simulink model "Discrete_Time_Sim_With_Noise"  (R2024b)
settings: Solver=FixedStepAuto  StartTime=0.0  StopTime=10  FixedStep=0.001  RelTol=1e-3
undefined symbols (not defined in the file or in its folder): DiscIntNeverNeededParam, dspblkCoreblockFVToolHelper, gcbh
libraries: simulink x12, sharedTrackingLibrary x1
(part 3 of 4)

== matlab function Discrete_Time_Sim_With_Noise/PLANT/MATLAB Function ==
  data: F1 input; D2_THETA_1 output; F2 input; F3 input; F4 input; F5 input; F6 input; states input; D2_THETA_2 output; D2_THETA_3 output
function [D2_THETA_1, D2_THETA_2, D2_THETA_3]  = fcn(F1, F2, F3, F4, F5, F6, states)

theta1 = states(1);
theta2 = states(2);
theta3 = states(3);
D_THETA_1 = states(4);
D_THETA_2 = states(5);
D_THETA_3 = states(6);

D2_THETA_1 =  (-1.539e-5*(D_THETA_1^2)*sin(theta3) - 1.71e-5*(D_THETA_1^2)*sin(theta2 + theta3) - 3.078e-5*D_THETA_1*D_THETA_2*sin(theta3) - 1.539e-5*(D_THETA_2^2)*sin(theta3) - 0.005*F5 + 0.005*F6 - 0.00167751*cos(theta1 + theta2 + theta3))*(3.63505644e-25*cos(theta2)^5*cos(theta3) - 3.68050943939915e-41*cos(theta2)^5*cos(theta2 + theta3) + 2.685902814e-25*cos(theta2)^5 + 1.24318930248e-25*cos(theta2)^4*cos(theta3)^2 + 2.0719821708e-25*cos(theta2)^4*cos(theta3)*cos(theta2 + theta3) + 1.2878109665982e-24*cos(theta2)^4*cos(theta3) - 2.09789038045752e-41*cos(theta2)^4*cos(theta2 + theta3)^2 - 1.83610739736e-25*cos(theta2)^4*cos(theta2 + theta3) + 8.8367645009889e-25*cos(theta2)^4 + 1.0629268536204e-26*cos(theta2)^3*cos(theta3)^3 + 4.724119349424e-26*cos(theta2)^3*cos(theta3)^2*cos(theta2 + theta3) - 6.16002601581253e-26*cos(theta2)^3*cos(theta3)^2 + 2.62451074968e-26*cos(theta2)^3*cos(theta3)*cos(theta2 + theta3)^2 + 3.74214304861488e-25*cos(theta2)^3*cos(theta3)*cos(theta2 + theta3) + 6.21384488024183e-26*cos(theta2)^3*cos(theta3) - 3.98599172286928e-42*cos(theta2)^3*cos(theta2 + theta3)^3 - 2.3650525378476e-25*cos(theta2)^3*cos(theta2 + theta3)^2 - 7.71987719826993e-25*cos(theta2)^3*cos(theta2 + theta3) + 8.38323515722335e-26*cos(theta2)^3 - 7.93473833908007e-43*cos(theta2)^2*cos(theta3)^4 + 2.01956102187876e-27*cos(theta2)^2*cos(theta3)^3*cos(theta2 + theta3) - 9.3695033763576e-26*cos(theta2)^2*cos(theta3)^3 - 2.86985925493723e-42*cos(theta2)^2*cos(theta3)^2*cos(theta2 + theta3)^2 - 2.15497046691621e-26*cos(theta2)^2*cos(theta3)^2*cos(theta2 + theta3) - 1.26819891173571e-24*cos(theta2)^2*cos(theta3)^2 - 4.986570424392e-27*cos(theta2)^2*cos(theta3)*cos(theta2 + theta3)^3 - 6.5637701594122e-26*cos(theta2)^2*cos(theta3)*cos(theta2 + theta3)^2 + 7.61401026222758e-26*cos(theta2)^2*cos(theta3)*cos(theta2 + theta3) - 3.74900859167102e-24*cos(theta2)^2*cos(theta3) - 2.52446142448388e-43*cos(theta2)^2*cos(theta2 + theta3)^4 - 7.66153010292696e-26*cos(theta2)^2*cos(theta2 + theta3)^3 - 6.31437319392806e-25*cos(theta2)^2*cos(theta2 + theta3)^2 - 8.91648455143469e-26*cos(theta2)^2*cos(theta2 + theta3) - 2.1155156940042e-24*cos(theta2)^2 - 3.01520056885046e-44*cos(theta2)*cos(theta3)^4*cos(theta2 + theta3) - 8.01092538678574e-27*cos(theta2)*cos(theta3)^4 - 3.83716594156965e-28*cos(theta2)*cos(theta3)^3*cos(theta2 + theta3)^2 + 1.37615273640096e-42*cos(theta2)*cos(theta3)^3*cos(theta2 + theta3) - 1.85496430166527e-25*cos(theta2)*cos(theta3)^3 - 1.70540708514206e-27*cos(theta2)*cos(theta3)^2*cos(theta2 + theta3)^3 - 1.51757959915666e-27*cos(theta2)*cos(theta3)^2*cos(theta2 + theta3)^2 + 8.67876276633391e-26*cos(theta2)*cos(theta3)^2*cos(theta2 + theta3) - 1.36365086623514e-24*cos(theta2)*cos(theta3)^2 - 1.42117257095172e-27*cos(theta2)*cos(theta3)*cos(theta2 + theta3)^4 - 3.01373541426773e-26*cos(theta2)*cos(theta3)*cos(theta2 + theta3)^3 + 2.22036449911628e-26*cos(theta2)*cos(theta3)*cos(theta2 + theta3)^2 + 1.11057805596928e-24*cos(theta2)*cos(theta3)*cos(theta2 + theta3) - 3.26448649239842e-24*cos(theta2)*cos(theta3) - 1.02879873647463e-26*cos(theta2)*cos(theta2 + theta3)^4 - 1.3209536422709e-25*cos(theta2)*cos(theta2 + theta3)^3 - 4.29616849707247e-26*cos(theta2)*cos(theta2 + theta3)^2 + 2.65202956136331e-24*cos(theta2)*cos(theta2 + theta3) - 1.74004006107545e-24*cos(theta2) - 2.02575979005193e-59*cos(theta3)^5*cos(theta2 + theta3) + 5.98014779488668e-43*cos(theta3)^5 - 8.02043351314214e-44*cos(theta3)^4*cos(theta2 + theta3)^2 + 1.52207582348929e-27*cos(theta3)^4*cos(theta2 + theta3) + 1.95108227317459e-41*cos(theta3)^4 - 7.29061528898234e-29*cos(theta3)^3*cos(theta2 + theta3)^3 + 3.38239071886509e-27*cos(theta3)^3*cos(theta2 + theta3)^2 + 4.26646638968557e-26*cos(theta3)^3*cos(theta2 + theta3) + 1.8899235687627e-40*cos(theta3)^3 - 1.62013673088496e-28*cos(theta3)^2*cos(theta2 + theta3)^4 + 6.7088030292407e-29*cos(theta3)^2*cos(theta2 + theta3)^3 + 6.22716299696936e-26*cos(theta3)^2*cos(theta2 + theta3)^2 + 4.25432077327408e-25*cos(theta3)^2*cos(theta2 + theta3) + 6.09898516049535e-40*cos(theta3)^2 - 9.00075961602756e-29*cos(theta3)*cos(theta2 + theta3)^5 - 2.46812847229638e-27*cos(theta3)*cos(theta2 + theta3)^4 + 1.89624246399257e-27*cos(theta3)*cos(theta2 + theta3)^3 + 3.46349040793488e-25*cos(theta3)*cos(theta2 + theta3)^2 + 1.76046632262571e-24*cos(theta3)*cos(theta2 + theta3) + 6.40478913692262e-40*cos(theta3) - 5.05305803005056e-28*cos(theta2 + theta3)^5 - 8.74991172989347e-27*cos(theta2 + theta3)^4 - 4.36886312193583e-27*cos(theta2 + theta3)^3 + 5.8025573321258e-25*cos(theta2 + theta3)^2 + 2.5119375317781e-24*cos(theta2 + theta3) + 1.44945219916276e-40)/(-2.4173125326e-29*cos(theta2)^6 + 1.68480351534995e-45*cos(theta2)^5*cos(theta3)^2 + 1.24318930248e-29*cos(theta2)^5*cos(theta3)*cos(theta2 + theta3) - 8.267208861492e-30*cos(theta2)^5*cos(theta3) - 1.837157524776e-29*cos(theta2)^5*cos(theta2 + theta3) - 7.95308805089001e-29*cos(theta2)^5 + 4.96910304784844e-46*cos(theta2)^4*cos(theta3)^3 + 4.2517074144816e-30*cos(theta2)^4*cos(theta3)^2*cos(theta2 + theta3) - 1.30351402739176e-29*cos(theta2)^4*cos(theta3)^2 + 9.448238698848e-30*cos(theta2)^4*cos(theta3)*cos(theta2 + theta3)^2 + 3.6189286639241e-29*cos(theta2)^4*cos(theta3)*cos(theta2 + theta3) + 4.61869822034009e-30*cos(theta2)^4*cos(theta3) - 1.18662418921716e-29*cos(theta2)^4*cos(theta2 + theta3)^2 - 4.53326018900731e-29*cos(theta2)^4*cos(theta2 + theta3) + 4.3594677937059e-29*cos(theta2)^4 + 3.57063225258603e-47*cos(theta2)^3*cos(theta3)^4 + 3.63520983938177e-31*cos(theta2)^3*cos(theta3)^3*cos(theta2 + theta3) - 4.21627651936092e-30*cos(theta2)^3*cos(theta3)^3 + 2.42347322625451e-30*cos(theta2)^3*cos(theta3)^2*cos(theta2 + theta3)^2 - 1.20134355055852e-29*cos(theta2)^3*cos(theta3)^2*cos(theta2 + theta3) - 3.43300293142612e-29*cos(theta2)^3*cos(theta3)^2 + 2.69274802917168e-30*cos(theta2)^3*cos(theta3)*cos(theta2 + theta3)^3 + 2.0150993536043e-29*cos(theta2)^3*cos(theta3)*cos(theta2 + theta3)^2 + 5.63534559650117e-30*cos(theta2)^3*cos(theta3)*cos(theta2 + theta3) + 9.7221157676726e-29*cos(theta2)^3*cos(theta3) - 5.70227450582974e-30*cos(theta2)^3*cos(theta2 + theta3)^3 - 3.04273787272693e-29*cos(theta2)^3*cos(theta2 + theta3)^2 + 3.59990216559352e-29*cos(theta2)^3*cos(theta2 + theta3) + 3.58648408559206e-28*cos(theta2)^3 + 1.89957635837577e-47*cos(theta2)^2*cos(theta3)^4*cos(theta2 + theta3) - 3.60491642405359e-31*cos(theta2)^2*cos(theta3)^4 + 1.38137973896507e-31*cos(theta2)^2*cos(theta3)^3*cos(theta2 + theta3)^2 - 5.60764777075002e-30*cos(theta2)^2*cos(theta3)^3*cos(theta2 + theta3) + 2.88826263059469e-30*cos(theta2)^2*cos(theta3)^3 + 4.60459912988358e-31*cos(theta2)^2*cos(theta3)^2*cos(theta2 + theta3)^3 - 3.79232906893446e-30*cos(theta2)^2*cos(theta3)^2*cos(theta2 + theta3)^2 - 6.29405194904902e-29*cos(theta2)^2*cos(theta3)^2*cos(theta2 + theta3) + 9.58935468786729e-30*cos(theta2)^2*cos(theta3)^2 + 3.41081417028413e-31*cos(theta2)^2*cos(theta3)*cos(theta2 + theta3)^4 + 3.08041897367519e-30*cos(theta2)^2*cos(theta3)*cos(theta2 + theta3)^3 + 2.90806924984375e-30*cos(theta2)^2*cos(theta3)*cos(theta2 + theta3)^2 - 7.28000339594151e-29*cos(theta2)^2*cos(theta3)*cos(theta2 + theta3) + 7.20879423926059e-29*cos(theta2)^2*cos(theta3) - 1.46763494088099e-30*cos(theta2)^2*cos(theta2 + theta3)^4 - 1.29795873992592e-29*cos(theta2)^2*cos(theta2 + theta3)^3 + 8.73500231364621e-30*cos(theta2)^2*cos(theta2 + theta3)^2 + 1.32078956143804e-28*cos(theta2)^2*cos(theta2 + theta3) + 1.72565285236144e-28*cos(theta2)^2 + 9.11591905523368e-64*cos(theta2)*cos(theta3)^5*cos(theta2 + theta3) - 2.69106650769901e-47*cos(theta2)*cos(theta3)^5 + 1.26321827831989e-47*cos(theta2)*cos(theta3)^4*cos(theta2 + theta3)^2 - 4.10960472342109e-31*cos(theta2)*cos(theta3)^4*cos(theta2 + theta3) + 3.17766707009168e-30*cos(theta2)*cos(theta3)^4 + 1.31231075201682e-32*cos(theta2)*cos(theta3)^3*cos(theta2 + theta3)^3 - 1.0654530764425e-30*cos(theta2)*cos(theta3)^3*cos(theta2 + theta3)^2 - 5.24643811206926e-30*cos(theta2)*cos(theta3)^3*cos(theta2 + theta3) + 4.06630232008378e-29*cos(theta2)*cos(theta3)^3 + 2.91624611559293e-32*cos(theta2)*cos(theta3)^2*cos(theta2 + theta3)^4 - 4.97662089495417e-31*cos(theta2)*cos(theta3)^2*cos(theta2 + theta3)^3 - 1.047463027015e-29*cos(theta2)*cos(theta3)^2*cos(theta2 + theta3)^2 - 4.29929048438523e-29*cos(theta2)*cos(theta3)^2*cos(theta2 + theta3) + 8.39207365825604e-29*cos(theta2)*cos(theta3)^2 + 1.62013673088496e-32*cos(theta2)*cos(theta3)*cos(theta2 + theta3)^5 + 3.4965424579252e-32*cos(theta2)*cos(theta3)*cos(theta2 + theta3)^4 + 6.21476991212799e-31*cos(theta2)*cos(theta3)*cos(theta2 + theta3)^3 + 5.15887830478587e-30*cos(theta2)*cos(theta3)*cos(theta2 + theta3)^2 - 8.42520199308358e-29*cos(theta2)*cos(theta3)*cos(theta2 + theta3) - 1.6867624438866e-28*cos(theta2)*cos(theta3) - 1.8191008908182e-31*cos(theta2)*cos(theta2 + theta3)^5 - 2.36247616707124e-30*cos(theta2)*cos(theta2 + theta3)^4 + 6.16670417728925e-31*cos(theta2)*cos(theta2 + theta3)^3 + 7.04447071666353e-29*cos(theta2)*cos(theta2 + theta3)^2 + 6.06543830095423e-30*cos(theta2)*cos(theta2 + theta3) - 4.02794188138399e-28*cos(theta2) + 1.38561969639552e-64*cos(theta3)^5*cos(theta2 + theta3)^2 - 1.32938685480331e-47*cos(theta3)^5*cos(theta2 + theta3) + 2.71690534492839e-31*cos(theta3)^5 + 1.95927732963902e-49*cos(theta3)^4*cos(theta2 + theta3)^3 - 1.30137482908335e-32*cos(theta3)^4*cos(theta2 + theta3)^2 + 6.03756743317419e-31*cos(theta3)^4*cos(theta2 + theta3) + 6.09036231194474e-30*cos(theta3)^4 + 1.0844025294549e-48*cos(theta3)^3*cos(theta2 + theta3)^4 - 2.89194406462966e-32*cos(theta3)^3*cos(theta2 + theta3)^3 + 2.31154131989653e-31*cos(theta3)^3*cos(theta2 + theta3)^2 + 7.72597440815918e-30*cos(theta3)^3*cos(theta2 + theta3) + 4.06211054992354e-29*cos(theta3)^3 + 1.61303439560337e-48*cos(theta3)^2*cos(theta2 + theta3)^5 - 2.30653465920323e-32*cos(theta3)^2*cos(theta2 + theta3)^4 + 4.65033312116703e-32*cos(theta3)^2*cos(theta2 + theta3)^3 + 3.1905625621327e-30*cos(theta3)^2*cos(theta2 + theta3)^2 + 1.59449399506865e-29*cos(theta3)^2*cos(theta2 + theta3) + 5.46041136575185e-29*cos(theta3)^2 + 7.22254206986584e-49*cos(theta3)*cos(theta2 + theta3)^6 - 1.55533126164956e-32*cos(theta3)*cos(theta2 + theta3)^5 + 4.57330301497445e-32*cos(theta3)*cos(theta2 + theta3)^4 + 4.27510802434887e-30*cos(theta3)*cos(theta2 + theta3)^3 + 2.21000322234703e-29*cos(theta3)*cos(theta2 + theta3)^2 - 3.20484864338455e-29*cos(theta3)*cos(theta2 + theta3) - 1.73177378730269e-28*cos(theta3) - 8.64072923138647e-33*cos(theta2 + theta3)^6 - 1.49623490581178e-31*cos(theta2 + theta3)^5 - 8.06193485042738e-33*cos(theta2 + theta3)^4 + 1.1076413479177e-29*cos(theta2 + theta3)^3 + 4.35303484319962e-29*cos(theta2 + theta3)^2 - 7.65308957462958e-29*cos(theta2 + theta3) - 3.31303627628766e-28) + (-9.0e-5*(D_THETA_1^2)*sin(theta2) - 1.71e-5*(D_THETA_1^2)*sin(theta2 + theta3) + 3.078e-5*D_THETA_1*D_THETA_3*sin(theta3) + 3.078e-5*D_THETA_2*D_THETA_3*sin(theta3) + 1.539e-5*(D_THETA_3^2)*sin(theta3) - 0.005*F3 + 0.005*F4 - 0.008829*cos(theta1 + theta2) - 0.00167751*cos(theta1 + theta2 + theta3))*(-2.685902814e-25*cos(theta2)^5 + 6.2159465124e-26*cos(theta2)^4*cos(theta3)^2 + 6.906607236e-26*cos(theta2)^4*cos(theta3)*cos(theta2 + theta3) - 9.18578762388e-26*cos(theta2)^4*cos(theta3) + 6.99296793485839e-42*cos(theta2)^4*cos(theta2 + theta3)^2 - 2.04128613864e-25*cos(theta2)^4*cos(theta2 + theta3) - 1.14152312024289e-24*cos(theta2)^4 + 2.1258537072408e-26*cos(theta2)^3*cos(theta3)^3 + 7.086179024136e-26*cos(theta2)^3*cos(theta3)^2*cos(theta2 + theta3) + 1.9665413003304e-25*cos(theta2)^3*cos(theta3)^2 + 5.24902149936e-26*cos(theta2)^3*cos(theta3)*cos(theta2 + theta3)^2 + 1.7487209771217e-25*cos(theta2)^3*cos(theta3)*cos(theta2 + theta3) - 3.68646920743583e-26*cos(theta2)^3*cos(theta3) + 2.65732781524619e-42*cos(theta2)^3*cos(theta2 + theta3)^3 - 5.817665495124e-26*cos(theta2)^3*cos(theta2 + theta3)^2 - 6.99659045865808e-25*cos(theta2)^3*cos(theta2 + theta3) - 9.32161743667168e-25*cos(theta2)^3 + 1.81760491969088e-27*cos(theta2)^2*cos(theta3)^4 + 1.41369271531513e-26*cos(theta2)^2*cos(theta3)^3*cos(theta2 + theta3) - 1.18766525665888e-26*cos(theta2)^2*cos(theta3)^3 + 2.69274802917168e-26*cos(theta2)^2*cos(theta3)^2*cos(theta2 + theta3)^2 + 1.00388804688789e-25*cos(theta2)^2*cos(theta3)^2*cos(theta2 + theta3) + 8.10917262741545e-26*cos(theta2)^2*cos(theta3)^2 + 1.4959711273176e-26*cos(theta2)^2*cos(theta3)*cos(theta2 + theta3)^3 + 1.19573511689261e-25*cos(theta2)^2*cos(theta3)*cos(theta2 + theta3)^2 - 9.20656920992465e-27*cos(theta2)^2*cos(theta3)*cos(theta2 + theta3) + 9.35170759248721e-25*cos(theta2)^2*cos(theta3) + 2.52446142448388e-43*cos(theta2)^2*cos(theta2 + theta3)^4 - 7.3690429604904e-27*cos(theta2)^2*cos(theta2 + theta3)^3 - 1.515517482989e-25*cos(theta2)^2*cos(theta2 + theta3)^2 - 5.15404047091562e-25*cos(theta2)^2*cos(theta2 + theta3) + 2.03503663649485e-24*cos(theta2)^2 + 1.99136488891557e-59*cos(theta2)*cos(theta3)^5 + 6.90689869482537e-28*cos(theta2)*cos(theta3)^4*cos(theta2 + theta3) - 1.60218507735715e-26*cos(theta2)*cos(theta3)^4 + 3.06973275325572e-27*cos(theta2)*cos(theta3)^3*cos(theta2 + theta3)^2 - 2.23151843903832e-26*cos(theta2)*cos(theta3)^3*cos(theta2 + theta3) - 1.99104462632765e-25*cos(theta2)*cos(theta3)^3 + 4.26351771285516e-27*cos(theta2)*cos(theta3)^2*cos(theta2 + theta3)^3 + 1.68501034991616e-26*cos(theta2)*cos(theta3)^2*cos(theta2 + theta3)^2 - 2.10142937245606e-25*cos(theta2)*cos(theta3)^2*cos(theta2 + theta3) - 2.90442132213305e-25*cos(theta2)*cos(theta3)^2 + 1.89489676126896e-27*cos(theta2)*cos(theta3)*cos(theta2 + theta3)^4 + 2.39790735672035e-26*cos(theta2)*cos(theta3)*cos(theta2 + theta3)^3 + 4.93949851881683e-28*cos(theta2)*cos(theta3)*cos(theta2 + theta3)^2 - 3.5694674390298e-25*cos(theta2)*cos(theta3)*cos(theta2 + theta3) + 1.76001351545894e-24*cos(theta2)*cos(theta3) - 3.50029540623296e-28*cos(theta2)*cos(theta2 + theta3)^4 - 1.31354180132991e-26*cos(theta2)*cos(theta2 + theta3)^3 - 9.4900421055639e-26*cos(theta2)*cos(theta2 + theta3)^2 + 3.71365940007247e-25*cos(theta2)*cos(theta2 + theta3) + 3.77093512731948e-24*cos(theta2) + 4.64039367546081e-44*cos(theta3)^5*cos(theta2 + theta3) - 1.36986824114036e-27*cos(theta3)^5 + 6.56155376008411e-29*cos(theta3)^4*cos(theta2 + theta3)^2 - 4.56622747046788e-27*cos(theta3)^4*cos(theta2 + theta3) - 3.07077091358558e-26*cos(theta3)^4 + 2.1871845866947e-28*cos(theta3)^3*cos(theta2 + theta3)^3 - 3.81113787651895e-27*cos(theta3)^3*cos(theta2 + theta3)^2 - 7.30741696318655e-26*cos(theta3)^3*cos(theta2 + theta3) - 2.048122966348e-25*cos(theta3)^3 + 2.43020509632744e-28*cos(theta3)^2*cos(theta2 + theta3)^4 + 9.26334493472043e-28*cos(theta3)^2*cos(theta2 + theta3)^3 - 4.28545693951622e-26*cos(theta3)^2*cos(theta2 + theta3)^2 - 3.14277669705205e-25*cos(theta3)^2*cos(theta2 + theta3) - 2.75314858777404e-25*cos(theta3)^2 + 9.00075961602757e-29*cos(theta3)*cos(theta2 + theta3)^5 + 1.55857802688727e-27*cos(theta3)*cos(theta2 + theta3)^4 + 1.73352697397771e-28*cos(theta3)*cos(theta2 + theta3)^3 - 1.01579545750445e-25*cos(theta3)*cos(theta2 + theta3)^2 - 2.85849865618501e-25*cos(theta3)*cos(theta2 + theta3) + 8.73163254102196e-25*cos(theta3) - 3.36028358998364e-28*cos(theta2 + theta3)^4 - 5.81869130037915e-27*cos(theta2 + theta3)^3 - 2.90529397608726e-27*cos(theta2 + theta3)^2 + 3.85870062586365e-25*cos(theta2 + theta3) + 1.67043845863244e-24)/(-2.4173125326e-29*cos(theta2)^6 + 1.68480351534995e-45*cos(theta2)^5*cos(theta3)^2 + 1.24318930248e-29*cos(theta2)^5*cos(theta3)*cos(theta2 + theta3) - 8.267208861492e-30*cos(theta2)^5*cos(theta3) - 1.837157524776e-29*cos(theta2)^5*cos(theta2 + theta3) - 7.95308805089001e-29*cos(theta2)^5 + 4.96910304784844e-46*cos(theta2)^4*cos(theta3)^3 + 4.2517074144816e-30*cos(theta2)^4*cos(theta3)^2*cos(theta2 + theta3) - 1.30351402739176e-29*cos(theta2)^4*cos(theta3)^2 + 9.448238698848e-30*cos(theta2)^4*cos(theta3)*cos(theta2 + theta3)^2 + 3.6189286639241e-29*cos(theta2)^4*cos(theta3)*cos(theta2 + theta3) + 4.61869822034009e-30*cos(theta2)^4*cos(theta3) - 1.18662418921716e-29*cos(theta2)^4*cos(theta2 + theta3)^2 - 4.53326018900731e-29*cos(theta2)^4*cos(theta2 + theta3) + 4.3594677937059e-29*cos(theta2)^4 + 3.57063225258603e-47*cos(theta2)^3*cos(theta3)^4 + 3.63520983938177e-31*cos(theta2)^3*cos(theta3)^3*cos(theta2 + theta3) - 4.21627651936092e-30*cos(theta2)^3*cos(theta3)^3 + 2.42347322625451e-30*cos(theta2)^3*cos(theta3)^2*cos(theta2 + theta3)^2 - 1.20134355055852e-29*cos(theta2)^3*cos(theta3)^2*cos(theta2 + theta3) - 3.43300293142612e-29*cos(theta2)^3*cos(theta3)^2 + 2.69274802917168e-30*cos(theta2)^3*cos(theta3)*cos(theta2 + theta3)^3 + 2.0150993536043e-29*cos(theta2)^3*cos(theta3)*cos(theta2 + theta3)^2 + 5.63534559650117e-30*cos(theta2)^3*cos(theta3)*cos(theta2 + theta3) + 9.7221157676726e-29*cos(theta2)^3*cos(theta3) - 5.70227450582974e-30*cos(theta2)^3*cos(theta2 + theta3)^3 - 3.04273787272693e-29*cos(theta2)^3*cos(theta2 + theta3)^2 + 3.59990216559352e-29*cos(theta2)^3*cos(theta2 + theta3) + 3.58648408559206e-28*cos(theta2)^3 + 1.89957635837577e-47*cos(theta2)^2*cos(theta3)^4*cos(theta2 + theta3) - 3.60491642405359e-31*cos(theta2)^2*cos(theta3)^4 + 1.38137973896507e-31*cos(theta2)^2*cos(theta3)^3*cos(theta2 + theta3)^2 - 5.60764777075002e-30*cos(theta2)^2*cos(theta3)^3*cos(theta2 + theta3) + 2.88826263059469e-30*cos(theta2)^2*cos(theta3)^3 + 4.60459912988358e-31*cos(theta2)^2*cos(theta3)^2*cos(theta2 + theta3)^3 - 3.79232906893446e-30*cos(theta2)^2*cos(theta3)^2*cos(theta2 + theta3)^2 - 6.29405194904902e-29*cos(theta2)^2*cos(theta3)^2*cos(theta2 + theta3) + 9.58935468786729e-30*cos(theta2)^2*cos(theta3)^2 + 3.41081417028413e-31*cos(theta2)^2*cos(theta3)*cos(theta2 + theta3)^4 + 3.08041897367519e-30*cos(theta2)^2*cos(theta3)*cos(theta2 + theta3)^3 + 2.90806924984375e-30*cos(theta2)^2*cos(theta3)*cos(theta2 + theta3)^2 - 7.28000339594151e-29*cos(theta2)^2*cos(theta3)*cos(theta2 + theta3) + 7.20879423926059e-29*cos(theta2)^2*cos(theta3) - 1.46763494088099e-30*cos(theta2)^2*cos(theta2 + theta3)^4 - 1.29795873992592e-29*cos(theta2)^2*cos(theta2 + theta3)^3 + 8.73500231364621e-30*cos(theta2)^2*cos(theta2 + theta3)^2 + 1.32078956143804e-28*cos(theta2)^2*cos(theta2 + theta3) + 1.72565285236144e-28*cos(theta2)^2 + 9.11591905523368e-64*cos(theta2)*cos(theta3)^5*cos(theta2 + theta3) - 2.69106650769901e-47*cos(theta2)*cos(theta3)^5 + 1.26321827831989e-47*cos(theta2)*cos(theta3)^4*cos(theta2 + theta3)^2 - 4.10960472342109e-31*cos(theta2)*cos(theta3)^4*cos(theta2 + theta3) + 3.17766707009168e-30*cos(theta2)*cos(theta3)^4 + 1.31231075201682e-32*cos(theta2)*cos(theta3)^3*cos(theta2 + theta3)^3 - 1.0654530764425e-30*cos(theta2)*cos(theta3)^3*cos(theta2 + theta3)^2 - 5.24643811206926e-30*cos(theta2)*cos(theta3)^3*cos(theta2 + theta3) + 4.06630232008378e-29*cos(theta2)*cos(theta3)^3 + 2.91624611559293e-32*cos(theta2)*cos(theta3)^2*cos(theta2 + theta3)^4 - 4.97662089495417e-31*cos(theta2)*cos(theta3)^2*cos(theta2 + theta3)^3 - 1.047463027015e-29*cos(theta2)*cos(theta3)^2*cos(theta2 + theta3)^2 - 4.29929048438523e-29*cos(theta2)*cos(theta3)^2*cos(theta2 + theta3) + 8.39207365825604e-29*cos(theta2)*cos(theta3)^2 + 1.62013673088496e-32*cos(theta2)*cos(theta3)*cos(theta2 + theta3)^5 + 3.4965424579252e-32*cos(theta2)*cos(theta3)*cos(theta2 + theta3)^4 + 6.21476991212799e-31*cos(theta2)*cos(theta3)*cos(theta2 + theta3)^3 + 5.15887830478587e-30*cos(theta2)*cos(theta3)*cos(theta2 + theta3)^2 - 8.42520199308358e-29*cos(theta2)*cos(theta3)*cos(theta2 + theta3) - 1.6867624438866e-28*cos(theta2)*cos(theta3) - 1.8191008908182e-31*cos(theta2)*cos(theta2 + theta3)^5 - 2.36247616707124e-30*cos(theta2)*cos(theta2 + theta3)^4 + 6.16670417728925e-31*cos(theta2)*cos(theta2 + theta3)^3 + 7.04447071666353e-29*cos(theta2)*cos(theta2 + theta3)^2 + 6.06543830095423e-30*cos(theta2)*cos(theta2 + theta3) - 4.02794188138399e-28*cos(theta2) + 1.38561969639552e-64*cos(theta3)^5*cos(theta2 + theta3)^2 - 1.32938685480331e-47*cos(theta3)^5*cos(theta2 + theta3) + 2.71690534492839e-31*cos(theta3)^5 + 1.95927732963902e-49*cos(theta3)^4*cos(theta2 + theta3)^3 - 1.30137482908335e-32*cos(theta3)^4*cos(theta2 + theta3)^2 + 6.03756743317419e-31*cos(theta3)^4*cos(theta2 + theta3) + 6.09036231194474e-30*cos(theta3)^4 + 1.0844025294549e-48*cos(theta3)^3*cos(theta2 + theta3)^4 - 2.89194406462966e-32*cos(theta3)^3*cos(theta2 + theta3)^3 + 2.31154131989653e-31*cos(theta3)^3*cos(theta2 + theta3)^2 + 7.72597440815918e-30*cos(theta3)^3*cos(theta2 + theta3) + 4.06211054992354e-29*cos(theta3)^3 + 1.61303439560337e-48*cos(theta3)^2*cos(theta2 + theta3)^5 - 2.30653465920323e-32*cos(theta3)^2*cos(theta2 + theta3)^4 + 4.65033312116703e-32*cos(theta3)^2*cos(theta2 + theta3)^3 + 3.1905625621327e-30*cos(theta3)^2*cos(theta2 + theta3)^2 + 1.59449399506865e-29*cos(theta3)^2*cos(theta2 + theta3) + 5.46041136575185e-29*cos(theta3)^2 + 7.22254206986584e-49*cos(theta3)*cos(theta2 + theta3)^6 - 1.55533126164956e-32*cos(theta3)*cos(theta2 + theta3)^5 + 4.57330301497445e-32*cos(theta3)*cos(theta2 + theta3)^4 + 4.27510802434887e-30*cos(theta3)*cos(theta2 + theta3)^3 + 2.21000322234703e-29*cos(theta3)*cos(theta2 + theta3)^2 - 3.20484864338455e-29*cos(theta3)*cos(theta2 + theta3) - 1.73177378730269e-28*cos(theta3) - 8.64072923138647e-33*cos(theta2 + theta3)^6 - 1.49623490581178e-31*cos(theta2 + theta3)^5 - 8.06193485042738e-33*cos(theta2 + theta3)^4 + 1.1076413479177e-29*cos(theta2 + theta3)^3 + 4.35303484319962e-29*cos(theta2 + theta3)^2 - 7.65308957462958e-29*cos(theta2 + theta3) - 3.31303627628766e-28) + (0.00018*D_THETA_1*D_THETA_2*sin(theta2) + 3.42e-5*D_THETA_1*D_THETA_2*sin(theta2 + theta3) + 3.078e-5*D_THETA_1*D_THETA_3*sin(theta3) + 3.42e-5*D_THETA_1*D_THETA_3*sin(theta2 + theta3) + 9.0e-5*(D_THETA_2^2)*sin(theta2) + 1.71e-5*(D_THETA_2^2)*sin(theta2 + theta3) + 3.078e-5*D_THETA_2*D_THETA_3*sin(theta3) + 3.42e-5*D_THETA_2*D_THETA_3*sin(theta2 + theta3) + 1.539e-5*(D_THETA_3^2)*sin(theta3) + 1.71e-5*(D_THETA_3^2)*sin(theta2 + theta3) - 0.005*F1 + 0.005*F2 - 0.018639*cos(theta1) - 0.008829*cos(theta1 + theta2) - 0.00167751*cos(theta1 + theta2 + theta3))*(-6.2159465124e-26*cos(theta2)^4*cos(theta3)^2 + 1.25873422827451e-41*cos(theta2)^4*cos(theta3)*cos(theta2 + theta3) + 1.14794370197489e-41*cos(theta2)^4*cos(theta3) - 6.37236764452981e-58*cos(theta2)^4*cos(theta2 + theta3)^2 + 9.30064735336166e-42*cos(theta2)^4*cos(theta2 + theta3) + 2.57846670144e-25*cos(theta2)^4 - 2.1258537072408e-26*cos(theta2)^3*cos(theta3)^3 - 4.724119349424e-26*cos(theta2)^3*cos(theta3)^2*cos(theta2 + theta3) - 2.04507978451457e-25*cos(theta2)^3*cos(theta3)^2 + 1.59309191113245e-58*cos(theta2)^3*cos(theta3)*cos(theta2 + theta3)^2 + 2.29588740394978e-41*cos(theta2)^3*cos(theta3)*cos(theta2 + theta3) + 8.81835611892481e-26*cos(theta2)^3*cos(theta3) - 1.16593754377894e-41*cos(theta2)^3*cos(theta2 + theta3)^2 + 1.9596346930944e-25*cos(theta2)^3*cos(theta2 + theta3) + 8.48329392094935e-25*cos(theta2)^3 - 1.81760491969088e-27*cos(theta2)^2*cos(theta3)^4 - 1.21173661312726e-26*cos(theta2)^2*cos(theta3)^3*cos(theta2 + theta3) + 1.18766525665888e-26*cos(theta2)^2*cos(theta3)^3 - 1.34637401458584e-26*cos(theta2)^2*cos(theta3)^2*cos(theta2 + theta3)^2 - 1.16569547717331e-25*cos(theta2)^2*cos(theta3)^2*cos(theta2 + theta3) - 1.1861506882179e-26*cos(theta2)^2*cos(theta3)^2 - 4.54403056407098e-43*cos(theta2)^2*cos(theta3)*cos(theta2 + theta3)^3 - 1.14794370197489e-41*cos(theta2)^2*cos(theta3)*cos(theta2 + theta3)^2 + 5.02646298778714e-26*cos(theta2)^2*cos(theta3)*cos(theta2 + theta3) - 4.92661143502941e-26*cos(theta2)^2*cos(theta3) - 2.55103470263634e-42*cos(theta2)^2*cos(theta2 + theta3)^3 + 5.58495887531904e-26*cos(theta2)^2*cos(theta2 + theta3)^2 + 4.83547753494113e-25*cos(theta2)^2*cos(theta2 + theta3) + 8.04790575093442e-26*cos(theta2)^2 - 6.90689869482537e-28*cos(theta2)*cos(theta3)^4*cos(theta2 + theta3) + 1.60218507735715e-26*cos(theta2)*cos(theta3)^4 - 2.30229956494179e-27*cos(theta2)*cos(theta3)^3*cos(theta2 + theta3)^2 + 4.51312797530374e-27*cos(theta2)*cos(theta3)^3*cos(theta2 + theta3) + 2.05023646390779e-25*cos(theta2)*cos(theta3)^3 - 1.70540708514206e-27*cos(theta2)*cos(theta3)^2*cos(theta2 + theta3)^3 - 2.21482140662928e-26*cos(theta2)*cos(theta3)^2*cos(theta2 + theta3)^2 - 4.50737261522801e-27*cos(theta2)*cos(theta3)^2*cos(theta2 + theta3) + 4.23129764281817e-25*cos(theta2)*cos(theta3)^2 + 9.55027967679557e-27*cos(theta2)*cos(theta3)*cos(theta2 + theta3)^2 - 1.87211234531119e-26*cos(theta2)*cos(theta3)*cos(theta2 + theta3) - 8.5046845910249e-25*cos(theta2)*cos(theta3) + 7.07428124207079e-27*cos(theta2)*cos(theta2 + theta3)^3 + 9.18740731638814e-26*cos(theta2)*cos(theta2 + theta3)^2 + 3.05820418535508e-26*cos(theta2)*cos(theta2 + theta3) - 2.03089506624403e-24*cos(theta2) - 4.64039367546081e-44*cos(theta3)^5*cos(theta2 + theta3) + 1.36986824114036e-27*cos(theta3)^5 - 6.5615537600841e-29*cos(theta3)^4*cos(theta2 + theta3)^2 + 3.04415164697858e-27*cos(theta3)^4*cos(theta2 + theta3) + 3.07077091358558e-26*cos(theta3)^4 - 1.45812305779647e-28*cos(theta3)^3*cos(theta2 + theta3)^3 + 4.28747157653854e-28*cos(theta3)^3*cos(theta2 + theta3)^2 + 3.89544928142479e-26*cos(theta3)^3*cos(theta2 + theta3) + 2.048122966348e-25*cos(theta3)^3 - 8.10068365442481e-29*cos(theta3)^2*cos(theta2 + theta3)^4 - 1.40272022419855e-27*cos(theta3)^2*cos(theta2 + theta3)^3 - 4.28200398446673e-28*cos(theta3)^2*cos(theta2 + theta3)^2 + 8.03946552135452e-26*cos(theta3)^2*cos(theta2 + theta3) + 2.75314858777404e-25*cos(theta3)^2 + 1.79366203433577e-43*cos(theta3)*cos(theta2 + theta3)^4 + 6.04851046197053e-28*cos(theta3)*cos(theta2 + theta3)^3 - 1.7785067280456e-27*cos(theta3)*cos(theta2 + theta3)^2 - 1.61589007229473e-25*cos(theta3)*cos(theta2 + theta3) - 8.73163254102196e-25*cos(theta3) + 3.36028358998363e-28*cos(theta2 + theta3)^4 + 5.81869130037916e-27*cos(theta2 + theta3)^3 + 2.90529397608731e-27*cos(theta2 + theta3)^2 - 3.85870062586365e-25*cos(theta2 + theta3) - 1.67043845863244e-24)/(-2.4173125326e-29*cos(theta2)^6 + 1.68480351534995e-45*cos(theta2)^5*cos(theta3)^2 + 1.24318930248e-29*cos(theta2)^5*cos(theta3)*cos(theta2 + theta3) - 8.267208861492e-30*cos(theta2)^5*cos(theta3) - 1.837157524776e-29*cos(theta2)^5*cos(theta2 + theta3) - 7.95308805089001e-29*cos(theta2)^5 + 4.96910304784844e-46*cos(theta2)^4*cos(theta3)^3 + 4.2517074144816e-30*cos(theta2)^4*cos(theta3)^2*cos(theta2 + theta3) - 1.30351402739176e-29*cos(theta2)^4*cos(theta3)^2 + 9.448238698848e-30*cos(theta2)^4*cos(theta3)*cos(theta2 + theta3)^2 + 3.6189286639241e-29*cos(theta2)^4*cos(theta3)*cos(theta2 + theta3) + 4.61869822034009e-30*cos(theta2)^4*cos(theta3) - 1.18662418921716e-29*cos(theta2)^4*cos(theta2 + theta3)^2 - 4.53326018900731e-29*cos(theta2)^4*cos(theta2 + theta3) + 4.3594677937059e-29*cos(theta2)^4 + 3.57063225258603e-47*cos(theta2)^3*cos(theta3)^4 + 3.63520983938177e-31*cos(theta2)^3*cos(theta3)^3*cos(theta2 + theta3) - 4.21627651936092e-30*cos(theta2)^3*cos(theta3)^3 + 2.42347322625451e-30*cos(theta2)^3*cos(theta3)^2*cos(theta2 + theta3)^2 - 1.20134355055852e-29*cos(theta2)^3*cos(theta3)^2*cos(theta2 + theta3) - 3.43300293142612e-29*cos(theta2)^3*cos(theta3)^2 + 2.69274802917168e-30*cos(theta2)^3*cos(theta3)*cos(theta2 + theta3)^3 + 2.0150993536043e-29*cos(theta2)^3*cos(theta3)*cos(theta2 + theta3)^2 + 5.63534559650117e-30*cos(theta2)^3*cos(theta3)*cos(theta2 + theta3) + 9.7221157676726e-29*cos(theta2)^3*cos(theta3) - 5.70227450582974e-30*cos(theta2)^3*cos(theta2 + theta3)^3 - 3.04273787272693e-29*cos(theta2)^3*cos(theta2 + theta3)^2 + 3.59990216559352e-29*cos(theta2)^3*cos(theta2 + theta3) + 3.58648408559206e-28*cos(theta2)^3 + 1.89957635837577e-47*cos(theta2)^2*cos(theta3)^4*cos(theta2 + theta3) - 3.60491642405359e-31*cos(theta2)^2*cos(theta3)^4 + 1.38137973896507e-31*cos(theta2)^2*cos(theta3)^3*cos(theta2 + theta3)^2 - 5.60764777075002e-30*cos(theta2)^2*cos(theta3)^3*cos(theta2 + theta3) + 2.88826263059469e-30*cos(theta2)^2*cos(theta3)^3 + 4.60459912988358e-31*cos(theta2)^2*cos(theta3)^2*cos(theta2 + theta3)^3 - 3.79232906893446e-30*cos(theta2)^2*cos(theta3)^2*cos(theta2 + theta3)^2 - 6.29405194904902e-29*cos(theta2)^2*cos(theta3)^2*cos(theta2 + theta3) + 9.58935468786729e-30*cos(theta2)^2*cos(theta3)^2 + 3.41081417028413e-31*cos(theta2)^2*cos(theta3)*cos(theta2 + theta3)^4 + 3.08041897367519e-30*cos(theta2)^2*cos(theta3)*cos(theta2 + theta3)^3 + 2.90806924984375e-30*cos(theta2)^2*cos(theta3)*cos(theta2 + theta3)^2 - 7.28000339594151e-29*cos(theta2)^2*cos(theta3)*cos(theta2 + theta3) + 7.20879423926059e-29*cos(theta2)^2*cos(theta3) - 1.46763494088099e-30*cos(theta2)^2*cos(theta2 + theta3)^4 - 1.29795873992592e-29*cos(theta2)^2*cos(theta2 + theta3)^3 + 8.73500231364621e-30*cos(theta2)^2*cos(theta2 + theta3)^2 + 1.32078956143804e-28*cos(theta2)^2*cos(theta2 + theta3) + 1.72565285236144e-28*cos(theta2)^2 + 9.11591905523368e-64*cos(theta2)*cos(theta3)^5*cos(theta2 + theta3) - 2.69106650769901e-47*cos(theta2)*cos(theta3)^5 + 1.26321827831989e-47*cos(theta2)*cos(theta3)^4*cos(theta2 + theta3)^2 - 4.10960472342109e-31*cos(theta2)*cos(theta3)^4*cos(theta2 + theta3) + 3.17766707009168e-30*cos(theta2)*cos(theta3)^4 + 1.31231075201682e-32*cos(theta2)*cos(theta3)^3*cos(theta2 + theta3)^3 - 1.0654530764425e-30*cos(theta2)*cos(theta3)^3*cos(theta2 + theta3)^2 - 5.24643811206926e-30*cos(theta2)*cos(theta3)^3*cos(theta2 + theta3) + 4.06630232008378e-29*cos(theta2)*cos(theta3)^3 + 2.91624611559293e-32*cos(theta2)*cos(theta3)^2*cos(theta2 + theta3)^4 - 4.97662089495417e-31*cos(theta2)*cos(theta3)^2*cos(theta2 + theta3)^3 - 1.047463027015e-29*cos(theta2)*cos(theta3)^2*cos(theta2 + theta3)^2 - 4.29929048438523e-29*cos(theta2)*cos(theta3)^2*cos(theta2 + theta3) + 8.39207365825604e-29*cos(theta2)*cos(theta3)^2 + 1.62013673088496e-32*cos(theta2)*cos(theta3)*cos(theta2 + theta3)^5 + 3.4965424579252e-32*cos(theta2)*cos(theta3)*cos(theta2 + theta3)^4 + 6.21476991212799e-31*cos(theta2)*cos(theta3)*cos(theta2 + theta3)^3 + 5.15887830478587e-30*cos(theta2)*cos(theta3)*cos(theta2 + theta3)^2 - 8.42520199308358e-29*cos(theta2)*cos(theta3)*cos(theta2 + theta3) - 1.6867624438866e-28*cos(theta2)*cos(theta3) - 1.8191008908182e-31*cos(theta2)*cos(theta2 + theta3)^5 - 2.36247616707124e-30*cos(theta2)*cos(theta2 + theta3)^4 + 6.16670417728925e-31*cos(theta2)*cos(theta2 + theta3)^3 + 7.04447071666353e-29*cos(theta2)*cos(theta2 + theta3)^2 + 6.06543830095423e-30*cos(theta2)*cos(theta2 + theta3) - 4.02794188138399e-28*cos(theta2) + 1.38561969639552e-64*cos(theta3)^5*cos(theta2 + theta3)^2 - 1.32938685480331e-47*cos(theta3)^5*cos(theta2 + theta3) + 2.71690534492839e-31*cos(theta3)^5 + 1.95927732963902e-49*cos(theta3)^4*cos(theta2 + theta3)^3 - 1.30137482908335e-32*cos(theta3)^4*cos(theta2 + theta3)^2 + 6.03756743317419e-31*cos(theta3)^4*cos(theta2 + theta3) + 6.09036231194474e-30*cos(theta3)^4 + 1.0844025294549e-48*cos(theta3)^3*cos(theta2 + theta3)^4 - 2.89194406462966e-32*cos(theta3)^3*cos(theta2 + theta3)^3 + 2.31154131989653e-31*cos(theta3)^3*cos(theta2 + theta3)^2 + 7.72597440815918e-30*cos(theta3)^3*cos(theta2 + theta3) + 4.06211054992354e-29*cos(theta3)^3 + 1.61303439560337e-48*cos(theta3)^2*cos(theta2 + theta3)^5 - 2.30653465920323e-32*cos(theta3)^2*cos(theta2 + theta3)^4 + 4.65033312116703e-32*cos(theta3)^2*cos(theta2 + theta3)^3 + 3.1905625621327e-30*cos(theta3)^2*cos(theta2 + theta3)^2 + 1.59449399506865e-29*cos(theta3)^2*cos(theta2 + theta3) + 5.46041136575185e-29*cos(theta3)^2 + 7.22254206986584e-49*cos(theta3)*cos(theta2 + theta3)^6 - 1.55533126164956e-32*cos(theta3)*cos(theta2 + theta3)^5 + 4.57330301497445e-32*cos(theta3)*cos(theta2 + theta3)^4 + 4.27510802434887e-30*cos(theta3)*cos(theta2 + theta3)^3 + 2.21000322234703e-29*cos(theta3)*cos(theta2 + theta3)^2 - 3.20484864338455e-29*cos(theta3)*cos(theta2 + theta3) - 1.73177378730269e-28*cos(theta3) - 8.64072923138647e-33*cos(theta2 + theta3)^6 - 1.49623490581178e-31*cos(theta2 + theta3)^5 - 8.06193485042738e-33*cos(theta2 + theta3)^4 + 1.1076413479177e-29*cos(theta2 + theta3)^3 + 4.35303484319962e-29*cos(theta2 + theta3)^2 - 7.65308957462958e-29*cos(theta2 + theta3) - 3.31303627628766e-28) ;
D2_THETA_2 =  (-1.539e-5*(D_THETA_1^2)*sin(theta3) - 1.71e-5*(D_THETA_1^2)*sin(theta2 + theta3) - 3.078e-5*D_THETA_1*D_THETA_2*sin(theta3) - 1.539e-5*(D_THETA_2^2)*sin(theta3) - 0.005*F5 + 0.005*F6 - 0.00167751*cos(theta1 + theta2 + theta3))*(-2.0194758e-21*cos(theta2)^4*cos(theta3) + 2.243862e-21*cos(theta2)^4*cos(theta2 + theta3) - 1.49216823e-21*cos(theta2)^4 - 3.453303618e-22*cos(theta2)^3*cos(theta3)^2 - 3.83700402e-22*cos(theta2)^3*cos(theta3)*cos(theta2 + theta3) - 8.027578984995e-21*cos(theta2)^3*cos(theta3) + 1.70533512e-21*cos(theta2)^3*cos(theta2 + theta3)^2 + 4.99478487075e-21*cos(theta2)^3*cos(theta2 + theta3) - 5.74295346083025e-21*cos(theta2)^3 + 2.5778876995062e-38*cos(theta2)^2*cos(theta3)^3 - 6.56127687419999e-23*cos(theta2)^2*cos(theta3)^2*cos(theta2 + theta3) + 7.610057973e-22*cos(theta2)^2*cos(theta3)^2 + 2.1870922914e-22*cos(theta2)^2*cos(theta3)*cos(theta2 + theta3)^2 - 4.58761615502175e-21*cos(theta2)^2*cos(theta3)*cos(theta2 + theta3) - 1.9239955589925e-21*cos(theta2)^2*cos(theta3) + 4.860205092e-22*cos(theta2)^2*cos(theta2 + theta3)^3 + 3.1702310149455e-21*cos(theta2)^2*cos(theta2 + theta3)^2 - 4.63532505183949e-21*cos(theta2)^2*cos(theta2 + theta3) - 1.83709522317037e-21*cos(theta2)^2 + 9.79597325812365e-40*cos(theta2)*cos(theta3)^3*cos(theta2 + theta3) + 2.602639826766e-22*cos(theta2)*cos(theta3)^3 + 1.246642606098e-23*cos(theta2)*cos(theta3)^2*cos(theta2 + theta3)^2 - 5.78364405948e-22*cos(theta2)*cos(theta3)^2*cos(theta2 + theta3) + 6.87683734292142e-21*cos(theta2)*cos(theta3)^2 + 6.9257922561e-23*cos(theta2)*cos(theta3)*cos(theta2 + theta3)^3 - 8.73907334833306e-22*cos(theta2)*cos(theta3)*cos(theta2 + theta3)^2 - 8.10594406956285e-21*cos(theta2)*cos(theta3)*cos(theta2 + theta3) + 2.35462446511192e-20*cos(theta2)*cos(theta3) + 6.1562597832e-23*cos(theta2)*cos(theta2 + theta3)^4 + 6.22813456618785e-22*cos(theta2)*cos(theta2 + theta3)^3 - 1.13946165989109e-21*cos(theta2)*cos(theta2 + theta3)^2 - 1.53704820058556e-20*cos(theta2)*cos(theta2 + theta3) + 1.37485933623811e-20*cos(theta2) + 6.58141582213102e-55*cos(theta3)^4*cos(theta2 + theta3) - 1.94286802952784e-38*cos(theta3)^4 + 2.60572888666087e-39*cos(theta3)^3*cos(theta2 + theta3)^2 - 4.9450156708554e-23*cos(theta3)^3*cos(theta2 + theta3) + 5.73544702565099e-22*cos(theta3)^3 + 2.36862095158621e-24*cos(theta3)^2*cos(theta2 + theta3)^3 - 1.3736154641265e-22*cos(theta3)^2*cos(theta2 + theta3)^2 - 2.73132055186345e-22*cos(theta3)^2*cos(theta2 + theta3) + 7.76315177451386e-21*cos(theta3)^2 + 5.263602114636e-24*cos(theta3)*cos(theta2 + theta3)^4 - 5.54906146801237e-23*cos(theta3)*cos(theta2 + theta3)^3 - 1.47067313353731e-21*cos(theta3)*cos(theta2 + theta3)^2 - 2.56843940741033e-21*cos(theta3)*cos(theta2 + theta3) + 2.29491781074512e-20*cos(theta3) + 2.92422339702e-24*cos(theta2 + theta3)^5 + 4.00930551055292e-23*cos(theta2 + theta3)^4 - 8.85533987957364e-23*cos(theta2 + theta3)^3 - 2.85407244355612e-21*cos(theta2 + theta3)^2 - 6.98756038638342e-21*cos(theta2 + theta3) + 1.29499160281121e-20)/(-1.342951407e-25*cos(theta2)^5 + 9.36001952972197e-42*cos(theta2)^4*cos(theta3)^2 + 6.906607236e-26*cos(theta2)^4*cos(theta3)*cos(theta2 + theta3) - 2.29644690597e-26*cos(theta2)^4*cos(theta3) - 7.65482301990001e-26*cos(theta2)^4*cos(theta2 + theta3) - 2.20919112524723e-25*cos(theta2)^4 + 1.16004946477779e-42*cos(theta2)^3*cos(theta3)^3 + 1.181029837356e-26*cos(theta2)^3*cos(theta3)^2*cos(theta2 + theta3) - 6.8490521757e-26*cos(theta2)^3*cos(theta3)^2 + 3.93676612452e-26*cos(theta2)^3*cos(theta3)*cos(theta2 + theta3)^2 + 1.04889045341457e-25*cos(theta2)^3*cos(theta3)*cos(theta2 + theta3) + 1.012137710409e-25*cos(theta2)^3*cos(theta3) - 5.137940232981e-26*cos(theta2)^3*cos(theta2 + theta3)^2 - 8.39492627593946e-26*cos(theta2)^3*cos(theta2 + theta3) + 6.05610527396333e-25*cos(theta2)^3 + 6.17146315261784e-43*cos(theta2)^2*cos(theta3)^3*cos(theta2 + theta3) - 1.1711879220447e-26*cos(theta2)^2*cos(theta3)^3 + 4.4879133819528e-27*cos(theta2)^2*cos(theta3)^2*cos(theta2 + theta3)^2 - 9.109239393681e-26*cos(theta2)^2*cos(theta3)^2*cos(theta2 + theta3) - 9.53611925396146e-26*cos(theta2)^2*cos(theta3)^2 + 7.479855636588e-27*cos(theta2)^2*cos(theta3)*cos(theta2 + theta3)^3 + 3.60460634296872e-26*cos(theta2)^2*cos(theta3)*cos(theta2 + theta3)^2 - 1.461131130816e-25*cos(theta2)^2*cos(theta3)*cos(theta2 + theta3) + 2.70058771324239e-25*cos(theta2)^2*cos(theta3) - 2.19172163675013e-26*cos(theta2)^2*cos(theta2 + theta3)^3 - 6.85701365403521e-26*cos(theta2)^2*cos(theta2 + theta3)^2 + 2.23027355982263e-25*cos(theta2)^2*cos(theta2 + theta3) + 9.96245579331129e-25*cos(theta2)^2 + 2.96163711995896e-59*cos(theta2)*cos(theta3)^4*cos(theta2 + theta3) - 8.74290613287526e-43*cos(theta2)*cos(theta3)^4 + 4.10402299649086e-43*cos(theta2)*cos(theta3)^3*cos(theta2 + theta3)^2 - 1.33515423113096e-26*cos(theta2)*cos(theta3)^3*cos(theta2 + theta3) + 5.1619023230859e-26*cos(theta2)*cos(theta3)^3 + 4.26351771285517e-28*cos(theta2)*cos(theta3)^2*cos(theta2 + theta3)^3 - 1.73075548479939e-26*cos(theta2)*cos(theta3)^2*cos(theta2 + theta3)^2 - 1.56716149779946e-25*cos(theta2)*cos(theta3)^2*cos(theta2 + theta3) + 1.63965865166209e-25*cos(theta2)*cos(theta3)^2 + 4.7372419031724e-28*cos(theta2)*cos(theta3)*cos(theta2 + theta3)^4 + 1.7079673196794e-27*cos(theta2)*cos(theta3)*cos(theta2 + theta3)^3 - 3.65381713457648e-27*cos(theta2)*cos(theta3)*cos(theta2 + theta3)^2 - 2.53533483105536e-25*cos(theta2)*cos(theta3)*cos(theta2 + theta3) - 2.14123355624304e-25*cos(theta2)*cos(theta3) - 3.9892563395136e-27*cos(theta2)*cos(theta2 + theta3)^4 - 2.30260834997197e-26*cos(theta2)*cos(theta2 + theta3)^3 + 1.18952308838765e-25*cos(theta2)*cos(theta2 + theta3)^2 + 1.7759932921543e-25*cos(theta2)*cos(theta2 + theta3) - 6.80154699948721e-25*cos(theta2) + 4.50168842233762e-60*cos(theta3)^4*cos(theta2 + theta3)^2 - 4.31899562964038e-43*cos(theta3)^4*cos(theta2 + theta3) + 8.82685297247688e-27*cos(theta3)^4 + 6.36542342312871e-45*cos(theta3)^3*cos(theta2 + theta3)^3 - 4.22798839858138e-28*cos(theta3)^3*cos(theta2 + theta3)^2 + 9.80761441386321e-27*cos(theta3)^3*cos(theta2 + theta3) + 1.12952842224549e-25*cos(theta3)^3 + 2.81580587519136e-44*cos(theta3)^2*cos(theta2 + theta3)^4 - 4.69776488731264e-28*cos(theta3)^2*cos(theta2 + theta3)^3 + 6.79873263328515e-28*cos(theta3)^2*cos(theta2 + theta3)^2 + 3.11535143815798e-26*cos(theta3)^2*cos(theta2 + theta3) + 2.33113157173779e-25*cos(theta3)^2 + 2.11185440639352e-44*cos(theta3)*cos(theta2 + theta3)^5 - 2.27387611352275e-28*cos(theta3)*cos(theta2 + theta3)^4 + 5.27468338224576e-27*cos(theta3)*cos(theta2 + theta3)^3 + 6.2501579303346e-26*cos(theta3)*cos(theta2 + theta3)^2 - 4.06834375686178e-26*cos(theta3)*cos(theta2 + theta3) - 4.68545123301835e-25*cos(theta3) - 2.52652901502528e-28*cos(theta2 + theta3)^5 - 2.18747793247337e-27*cos(theta2 + theta3)^4 + 1.87035337358171e-26*cos(theta2 + theta3)^3 + 1.61935869578611e-25*cos(theta2 + theta3)^2 - 1.29229392990257e-25*cos(theta2 + theta3) - 1.11887274482889e-24) + (-9.0e-5*(D_THETA_1^2)*sin(theta2) - 1.71e-5*(D_THETA_1^2)*sin(theta2 + theta3) + 3.078e-5*D_THETA_1*D_THETA_3*sin(theta3) + 3.078e-5*D_THETA_2*D_THETA_3*sin(theta3) + 1.539e-5*(D_THETA_3^2)*sin(theta3) - 0.005*F3 + 0.005*F4 - 0.008829*cos(theta1 + theta2) - 0.00167751*cos(theta1 + theta2 + theta3))*(2.98433646e-21*cos(theta2)^4 - 3.453303618e-22*cos(theta2)^3*cos(theta3)^2 - 7.67400804e-22*cos(theta2)^3*cos(theta3)*cos(theta2 + theta3) + 5.1032153466e-22*cos(theta2)^3*cos(theta3) - 4.2633378e-22*cos(theta2)^3*cos(theta2 + theta3)^2 + 1.7010717822e-21*cos(theta2)^3*cos(theta2 + theta3) + 9.6300917674605e-21*cos(theta2)^3 - 5.90514918678e-23*cos(theta2)^2*cos(theta3)^3 - 3.2806384371e-22*cos(theta2)^2*cos(theta3)^2*cos(theta2 + theta3) - 5.68077717920715e-22*cos(theta2)^2*cos(theta3)^2 - 5.1032153466e-22*cos(theta2)^2*cos(theta3)*cos(theta2 + theta3)^2 - 1.0684727455419e-21*cos(theta2)^2*cos(theta3)*cos(theta2 + theta3) - 1.4419418473782e-21*cos(theta2)^2*cos(theta3) - 2.430102546e-22*cos(theta2)^2*cos(theta2 + theta3)^3 - 3.781268773335e-22*cos(theta2)^2*cos(theta2 + theta3)^2 + 4.55638272123699e-21*cos(theta2)^2*cos(theta2 + theta3) + 6.21324685608166e-22*cos(theta2)^2 - 2.2439566909764e-23*cos(theta2)*cos(theta3)^3*cos(theta2 + theta3) + 2.602639826766e-22*cos(theta2)*cos(theta3)^3 - 8.726498242686e-23*cos(theta2)*cos(theta3)^2*cos(theta2 + theta3)^2 + 3.62494873138128e-22*cos(theta2)*cos(theta3)^2*cos(theta2 + theta3) + 4.42106317941435e-22*cos(theta2)*cos(theta3)^2 - 1.108126760976e-22*cos(theta2)*cos(theta3)*cos(theta2 + theta3)^3 - 1.399739066496e-22*cos(theta2)*cos(theta3)*cos(theta2 + theta3)^2 + 1.71656168216198e-21*cos(theta2)*cos(theta3)*cos(theta2 + theta3) - 8.47958560841253e-21*cos(theta2)*cos(theta3) - 4.6171948374e-23*cos(theta2)*cos(theta2 + theta3)^4 - 2.4603603228243e-22*cos(theta2)*cos(theta2 + theta3)^3 + 1.70912680169958e-21*cos(theta2)*cos(theta2 + theta3)^2 + 1.59355498757162e-21*cos(theta2)*cos(theta2 + theta3) - 2.3054377274039e-20*cos(theta2) - 1.50760028442521e-39*cos(theta3)^4*cos(theta2 + theta3) + 4.45051410376986e-23*cos(theta3)^4 - 2.13175885642759e-24*cos(theta3)^3*cos(theta2 + theta3)^2 + 1.48350470125662e-22*cos(theta3)^3*cos(theta2 + theta3) + 5.69510128863274e-22*cos(theta3)^3 - 7.10586285475861e-24*cos(theta3)^2*cos(theta2 + theta3)^3 + 1.44326250078242e-22*cos(theta3)^2*cos(theta2 + theta3)^2 + 1.42265460724101e-21*cos(theta3)^2*cos(theta2 + theta3) + 7.51574648331947e-22*cos(theta3)^2 - 7.89540317195401e-24*cos(theta3)*cos(theta2 + theta3)^4 + 1.54771192568715e-23*cos(theta3)*cos(theta2 + theta3)^3 + 1.08129974482369e-21*cos(theta3)*cos(theta2 + theta3)^2 + 2.34616558116548e-21*cos(theta3)*cos(theta2 + theta3) - 7.78538835053741e-21*cos(theta3) - 2.92422339702e-24*cos(theta2 + theta3)^5 - 2.53180316258492e-23*cos(theta2 + theta3)^4 + 2.26301475519277e-22*cos(theta2 + theta3)^3 + 1.95932633601529e-21*cos(theta2 + theta3)^2 - 2.14728733839631e-21*cos(theta2 + theta3) - 1.85912912121233e-20)/(-1.342951407e-25*cos(theta2)^5 + 9.36001952972197e-42*cos(theta2)^4*cos(theta3)^2 + 6.906607236e-26*cos(theta2)^4*cos(theta3)*cos(theta2 + theta3) - 2.29644690597e-26*cos(theta2)^4*cos(theta3) - 7.65482301990001e-26*cos(theta2)^4*cos(theta2 + theta3) - 2.20919112524723e-25*cos(theta2)^4 + 1.16004946477779e-42*cos(theta2)^3*cos(theta3)^3 + 1.181029837356e-26*cos(theta2)^3*cos(theta3)^2*cos(theta2 + theta3) - 6.8490521757e-26*cos(theta2)^3*cos(theta3)^2 + 3.93676612452e-26*cos(theta2)^3*cos(theta3)*cos(theta2 + theta3)^2 + 1.04889045341457e-25*cos(theta2)^3*cos(theta3)*cos(theta2 + theta3) + 1.012137710409e-25*cos(theta2)^3*cos(theta3) - 5.137940232981e-26*cos(theta2)^3*cos(theta2 + theta3)^2 - 8.39492627593946e-26*cos(theta2)^3*cos(theta2 + theta3) + 6.05610527396333e-25*cos(theta2)^3 + 6.17146315261784e-43*cos(theta2)^2*cos(theta3)^3*cos(theta2 + theta3) - 1.1711879220447e-26*cos(theta2)^2*cos(theta3)^3 + 4.4879133819528e-27*cos(theta2)^2*cos(theta3)^2*cos(theta2 + theta3)^2 - 9.109239393681e-26*cos(theta2)^2*cos(theta3)^2*cos(theta2 + theta3) - 9.53611925396146e-26*cos(theta2)^2*cos(theta3)^2 + 7.479855636588e-27*cos(theta2)^2*cos(theta3)*cos(theta2 + theta3)^3 + 3.60460634296872e-26*cos(theta2)^2*cos(theta3)*cos(theta2 + theta3)^2 - 1.461131130816e-25*cos(theta2)^2*cos(theta3)*cos(theta2 + theta3) + 2.70058771324239e-25*cos(theta2)^2*cos(theta3) - 2.19172163675013e-26*cos(theta2)^2*cos(theta2 + theta3)^3 - 6.85701365403521e-26*cos(theta2)^2*cos(theta2 + theta3)^2 + 2.23027355982263e-25*cos(theta2)^2*cos(theta2 + theta3) + 9.96245579331129e-25*cos(theta2)^2 + 2.96163711995896e-59*cos(theta2)*cos(theta3)^4*cos(theta2 + theta3) - 8.74290613287526e-43*cos(theta2)*cos(theta3)^4 + 4.10402299649086e-43*cos(theta2)*cos(theta3)^3*cos(theta2 + theta3)^2 - 1.33515423113096e-26*cos(theta2)*cos(theta3)^3*cos(theta2 + theta3) + 5.1619023230859e-26*cos(theta2)*cos(theta3)^3 + 4.26351771285517e-28*cos(theta2)*cos(theta3)^2*cos(theta2 + theta3)^3 - 1.73075548479939e-26*cos(theta2)*cos(theta3)^2*cos(theta2 + theta3)^2 - 1.56716149779946e-25*cos(theta2)*cos(theta3)^2*cos(theta2 + theta3) + 1.63965865166209e-25*cos(theta2)*cos(theta3)^2 + 4.7372419031724e-28*cos(theta2)*cos(theta3)*cos(theta2 + theta3)^4 + 1.7079673196794e-27*cos(theta2)*cos(theta3)*cos(theta2 + theta3)^3 - 3.65381713457648e-27*cos(theta2)*cos(theta3)*cos(theta2 + theta3)^2 - 2.53533483105536e-25*cos(theta2)*cos(theta3)*cos(theta2 + theta3) - 2.14123355624304e-25*cos(theta2)*cos(theta3) - 3.9892563395136e-27*cos(theta2)*cos(theta2 + theta3)^4 - 2.30260834997197e-26*cos(theta2)*cos(theta2 + theta3)^3 + 1.18952308838765e-25*cos(theta2)*cos(theta2 + theta3)^2 + 1.7759932921543e-25*cos(theta2)*cos(theta2 + theta3) - 6.80154699948721e-25*cos(theta2) + 4.50168842233762e-60*cos(theta3)^4*cos(theta2 + theta3)^2 - 4.31899562964038e-43*cos(theta3)^4*cos(theta2 + theta3) + 8.82685297247688e-27*cos(theta3)^4 + 6.36542342312871e-45*cos(theta3)^3*cos(theta2 + theta3)^3 - 4.22798839858138e-28*cos(theta3)^3*cos(theta2 + theta3)^2 + 9.80761441386321e-27*cos(theta3)^3*cos(theta2 + theta3) + 1.12952842224549e-25*cos(theta3)^3 + 2.81580587519136e-44*cos(theta3)^2*cos(theta2 + theta3)^4 - 4.69776488731264e-28*cos(theta3)^2*cos(theta2 + theta3)^3 + 6.79873263328515e-28*cos(theta3)^2*cos(theta2 + theta3)^2 + 3.11535143815798e-26*cos(theta3)^2*cos(theta2 + theta3) + 2.33113157173779e-25*cos(theta3)^2 + 2.11185440639352e-44*cos(theta3)*cos(theta2 + theta3)^5 - 2.27387611352275e-28*cos(theta3)*cos(theta2 + theta3)^4 + 5.27468338224576e-27*cos(theta3)*cos(theta2 + theta3)^3 + 6.2501579303346e-26*cos(theta3)*cos(theta2 + theta3)^2 - 4.06834375686178e-26*cos(theta3)*cos(theta2 + theta3) - 4.68545123301835e-25*cos(theta3) - 2.52652901502528e-28*cos(theta2 + theta3)^5 - 2.18747793247337e-27*cos(theta2 + theta3)^4 + 1.87035337358171e-26*cos(theta2 + theta3)^3 + 1.61935869578611e-25*cos(theta2 + theta3)^2 - 1.29229392990257e-25*cos(theta2 + theta3) - 1.11887274482889e-24) + (0.00018*D_THETA_1*D_THETA_2*sin(theta2) + 3.42e-5*D_THETA_1*D_THETA_2*sin(theta2 + theta3) + 3.078e-5*D_THETA_1*D_THETA_3*sin(theta3) + 3.42e-5*D_THETA_1*D_THETA_3*sin(theta2 + theta3) + 9.0e-5*(D_THETA_2^2)*sin(theta2) + 1.71e-5*(D_THETA_2^2)*sin(theta2 + theta3) + 3.078e-5*D_THETA_2*D_THETA_3*sin(theta3) + 3.42e-5*D_THETA_2*D_THETA_3*sin(theta2 + theta3) + 1.539e-5*(D_THETA_3^2)*sin(theta3) + 1.71e-5*(D_THETA_3^2)*sin(theta2 + theta3) - 0.005*F1 + 0.005*F2 - 0.018639*cos(theta1) - 0.008829*cos(theta1 + theta2) - 0.00167751*cos(theta1 + theta2 + theta3))*(-1.49216823e-21*cos(theta2)^4 + 3.453303618e-22*cos(theta2)^3*cos(theta3)^2 + 3.83700402e-22*cos(theta2)^3*cos(theta3)*cos(theta2 + theta3) - 2.5516076733e-22*cos(theta2)^3*cos(theta3) + 3.88498218603244e-38*cos(theta2)^3*cos(theta2 + theta3)^2 - 8.50535891100001e-22*cos(theta2)^3*cos(theta2 + theta3) - 3.88713830663025e-21*cos(theta2)^3 + 5.90514918678e-23*cos(theta2)^2*cos(theta3)^3 + 2.62451074968e-22*cos(theta2)^2*cos(theta3)^2*cos(theta2 + theta3) + 5.68077717920715e-22*cos(theta2)^2*cos(theta3)^2 + 2.1870922914e-22*cos(theta2)^2*cos(theta3)*cos(theta2 + theta3)^2 + 5.3423637277095e-22*cos(theta2)^2*cos(theta3)*cos(theta2 + theta3) + 8.796431193732e-22*cos(theta2)^2*cos(theta3) + 7.38146615346164e-39*cos(theta2)^2*cos(theta2 + theta3)^3 - 1.61601819309e-22*cos(theta2)^2*cos(theta2 + theta3)^2 - 1.7492840416715e-21*cos(theta2)^2*cos(theta2 + theta3) + 1.21577053756221e-21*cos(theta2)^2 + 2.2439566909764e-23*cos(theta2)*cos(theta3)^3*cos(theta2 + theta3) - 2.602639826766e-22*cos(theta2)*cos(theta3)^3 + 6.23321303049e-23*cos(theta2)*cos(theta3)^2*cos(theta2 + theta3)^2 - 7.33126701641283e-23*cos(theta2)*cos(theta3)^2*cos(theta2 + theta3) - 6.34412482919145e-22*cos(theta2)*cos(theta3)^2 + 4.15547535366e-23*cos(theta2)*cos(theta3)*cos(theta2 + theta3)^3 + 2.306437327548e-22*cos(theta2)*cos(theta3)*cos(theta2 + theta3)^2 - 7.97985406721034e-22*cos(theta2)*cos(theta3)*cos(theta2 + theta3) + 3.54045979359856e-21*cos(theta2)*cos(theta3) - 1.023478188957e-23*cos(theta2)*cos(theta2 + theta3)^3 - 2.43750857227112e-22*cos(theta2)*cos(theta2 + theta3)^2 - 2.16732999246618e-22*cos(theta2)*cos(theta2 + theta3) + 9.30578391165787e-21*cos(theta2) + 1.50760028442521e-39*cos(theta3)^4*cos(theta2 + theta3) - 4.45051410376986e-23*cos(theta3)^4 + 2.13175885642758e-24*cos(theta3)^3*cos(theta2 + theta3)^2 - 9.89003134171079e-23*cos(theta3)^3*cos(theta2 + theta3) - 5.69510128863274e-22*cos(theta3)^3 + 4.7372419031724e-24*cos(theta3)^2*cos(theta2 + theta3)^3 - 3.44370129481222e-23*cos(theta3)^2*cos(theta2 + theta3)^2 - 7.89865575170707e-22*cos(theta3)^2*cos(theta2 + theta3) - 1.17536045633838e-21*cos(theta3)^2 + 2.631801057318e-24*cos(theta3)*cos(theta2 + theta3)^4 + 2.27862284632642e-23*cos(theta3)*cos(theta2 + theta3)^3 - 1.83372343886369e-22*cos(theta3)*cos(theta2 + theta3)^2 - 1.3059560625982e-21*cos(theta3)*cos(theta2 + theta3) + 2.3624123863958e-21*cos(theta3) - 9.82539061398724e-24*cos(theta2 + theta3)^3 - 8.5068586262853e-23*cos(theta2 + theta3)^2 + 6.51576771379448e-22*cos(theta2 + theta3) + 5.64137518401119e-21)/(-1.342951407e-25*cos(theta2)^5 + 9.36001952972197e-42*cos(theta2)^4*cos(theta3)^2 + 6.906607236e-26*cos(theta2)^4*cos(theta3)*cos(theta2 + theta3) - 2.29644690597e-26*cos(theta2)^4*cos(theta3) - 7.65482301990001e-26*cos(theta2)^4*cos(theta2 + theta3) - 2.20919112524723e-25*cos(theta2)^4 + 1.16004946477779e-42*cos(theta2)^3*cos(theta3)^3 + 1.181029837356e-26*cos(theta2)^3*cos(theta3)^2*cos(theta2 + theta3) - 6.8490521757e-26*cos(theta2)^3*cos(theta3)^2 + 3.93676612452e-26*cos(theta2)^3*cos(theta3)*cos(theta2 + theta3)^2 + 1.04889045341457e-25*cos(theta2)^3*cos(theta3)*cos(theta2 + theta3) + 1.012137710409e-25*cos(theta2)^3*cos(theta3) - 5.137940232981e-26*cos(theta2)^3*cos(theta2 + theta3)^2 - 8.39492627593946e-26*cos(theta2)^3*cos(theta2 + theta3) + 6.05610527396333e-25*cos(theta2)^3 + 6.17146315261784e-43*cos(theta2)^2*cos(theta3)^3*cos(theta2 + theta3) - 1.1711879220447e-26*cos(theta2)^2*cos(theta3)^3 + 4.4879133819528e-27*cos(theta2)^2*cos(theta3)^2*cos(theta2 + theta3)^2 - 9.109239393681e-26*cos(theta2)^2*cos(theta3)^2*cos(theta2 + theta3) - 9.53611925396146e-26*cos(theta2)^2*cos(theta3)^2 + 7.479855636588e-27*cos(theta2)^2*cos(theta3)*cos(theta2 + theta3)^3 + 3.60460634296872e-26*cos(theta2)^2*cos(theta3)*cos(theta2 + theta3)^2 - 1.461131130816e-25*cos(theta2)^2*cos(theta3)*cos(theta2 + theta3) + 2.70058771324239e-25*cos(theta2)^2*cos(theta3) - 2.19172163675013e-26*cos(theta2)^2*cos(theta2 + theta3)^3 - 6.85701365403521e-26*cos(theta2)^2*cos(theta2 + theta3)^2 + 2.23027355982263e-25*cos(theta2)^2*cos(theta2 + theta3) + 9.96245579331129e-25*cos(theta2)^2 + 2.96163711995896e-59*cos(theta2)*cos(theta3)^4*cos(theta2 + theta3) - 8.74290613287526e-43*cos(theta2)*cos(theta3)^4 + 4.10402299649086e-43*cos(theta2)*cos(theta3)^3*cos(theta2 + theta3)^2 - 1.33515423113096e-26*cos(theta2)*cos(theta3)^3*cos(theta2 + theta3) + 5.1619023230859e-26*cos(theta2)*cos(theta3)^3 + 4.26351771285517e-28*cos(theta2)*cos(theta3)^2*cos(theta2 + theta3)^3 - 1.73075548479939e-26*cos(theta2)*cos(theta3)^2*cos(theta2 + theta3)^2 - 1.56716149779946e-25*cos(theta2)*cos(theta3)^2*cos(theta2 + theta3) + 1.63965865166209e-25*cos(theta2)*cos(theta3)^2 + 4.7372419031724e-28*cos(theta2)*cos(theta3)*cos(theta2 + theta3)^4 + 1.7079673196794e-27*cos(theta2)*cos(theta3)*cos(theta2 + theta3)^3 - 3.65381713457648e-27*cos(theta2)*cos(theta3)*cos(theta2 + theta3)^2 - 2.53533483105536e-25*cos(theta2)*cos(theta3)*cos(theta2 + theta3) - 2.14123355624304e-25*cos(theta2)*cos(theta3) - 3.9892563395136e-27*cos(theta2)*cos(theta2 + theta3)^4 - 2.30260834997197e-26*cos(theta2)*cos(theta2 + theta3)^3 + 1.18952308838765e-25*cos(theta2)*cos(theta2 + theta3)^2 + 1.7759932921543e-25*cos(theta2)*cos(theta2 + theta3) - 6.80154699948721e-25*cos(theta2) + 4.50168842233762e-60*cos(theta3)^4*cos(theta2 + theta3)^2 - 4.31899562964038e-43*cos(theta3)^4*cos(theta2 + theta3) + 8.82685297247688e-27*cos(theta3)^4 + 6.36542342312871e-45*cos(theta3)^3*cos(theta2 + theta3)^3 - 4.22798839858138e-28*cos(theta3)^3*cos(theta2 + theta3)^2 + 9.80761441386321e-27*cos(theta3)^3*cos(theta2 + theta3) + 1.12952842224549e-25*cos(theta3)^3 + 2.81580587519136e-44*cos(theta3)^2*cos(theta2 + theta3)^4 - 4.69776488731264e-28*cos(theta3)^2*cos(theta2 + theta3)^3 + 6.79873263328515e-28*cos(theta3)^2*cos(theta2 + theta3)^2 + 3.11535143815798e-26*cos(theta3)^2*cos(theta2 + theta3) + 2.33113157173779e-25*cos(theta3)^2 + 2.11185440639352e-44*cos(theta3)*cos(theta2 + theta3)^5 - 2.27387611352275e-28*cos(theta3)*cos(theta2 + theta3)^4 + 5.27468338224576e-27*cos(theta3)*cos(theta2 + theta3)^3 + 6.2501579303346e-26*cos(theta3)*cos(theta2 + theta3)^2 - 4.06834375686178e-26*cos(theta3)*cos(theta2 + theta3) - 4.68545123301835e-25*cos(theta3) - 2.52652901502528e-28*cos(theta2 + theta3)^5 - 2.18747793247337e-27*cos(theta2 + theta3)^4 + 1.87035337358171e-26*cos(theta2 + theta3)^3 + 1.61935869578611e-25*cos(theta2 + theta3)^2 - 1.29229392990257e-25*cos(theta2 + theta3) - 1.11887274482889e-24) ;
D2_THETA_3 =  (-1.539e-5*(D_THETA_1^2)*sin(theta3) - 1.71e-5*(D_THETA_1^2)*sin(theta2 + theta3) - 3.078e-5*D_THETA_1*D_THETA_2*sin(theta3) - 1.539e-5*(D_THETA_2^2)*sin(theta3) - 0.005*F5 + 0.005*F6 - 0.00167751*cos(theta1 + theta2 + theta3))*(-1.458e-12*cos(theta2)^3 - 2.49317999999999e-13*cos(theta2)^2*cos(theta3) - 8.3106e-13*cos(theta2)^2*cos(theta2 + theta3) - 2.39844915e-12*cos(theta2)^2 - 9.47408400000007e-14*cos(theta2)*cos(theta3)*cos(theta2 + theta3) + 1.098846e-12*cos(theta2)*cos(theta3) - 1.579014e-13*cos(theta2)*cos(theta2 + theta3)^2 - 9.11410677e-13*cos(theta2)*cos(theta2 + theta3) + 3.49044255e-12*cos(theta2) - 6.36515481359555e-30*cos(theta3)^2*cos(theta2 + theta3) + 1.87902665999999e-13*cos(theta3)^2 - 9.00037980000001e-15*cos(theta3)*cos(theta2 + theta3)^2 + 2.08780739999999e-13*cos(theta3)*cos(theta2 + theta3) + 2.4044968521e-12*cos(theta3) - 1.0000422e-14*cos(theta2 + theta3)^3 - 8.6584014314999e-14*cos(theta2 + theta3)^2 + 6.631840845e-13*cos(theta2 + theta3) + 5.74187171959625e-12)/(-1.6579647e-17*cos(theta2)^3 + 1.15555796663234e-33*cos(theta2)^2*cos(theta3)^2 + 8.5266756e-18*cos(theta2)^2*cos(theta3)*cos(theta2 + theta3) - 2.835119637e-18*cos(theta2)^2*cos(theta3) - 3.15013293e-18*cos(theta2)^2*cos(theta2 + theta3) - 2.7273964509225e-17*cos(theta2)^2 + 1.432159833059e-34*cos(theta2)*cos(theta3)^3 + 1.4580615276e-18*cos(theta2)*cos(theta3)^2*cos(theta2 + theta3) - 8.45561997e-18*cos(theta2)*cos(theta3)^2 + 1.620068364e-18*cos(theta2)*cos(theta3)*cos(theta2 + theta3)^2 + 1.402661031903e-17*cos(theta2)*cos(theta3)*cos(theta2 + theta3) + 3.08148791101958e-33*cos(theta2)*cos(theta3) - 4.54756032e-18*cos(theta2)*cos(theta2 + theta3)^2 + 3.507516432e-17*cos(theta2) + 2.17688294624968e-35*cos(theta3)^3*cos(theta2 + theta3) - 1.44591101487e-18*cos(theta3)^3 + 9.62964972193618e-35*cos(theta3)^2*cos(theta2 + theta3)^2 - 1.6065677943e-18*cos(theta3)^2*cos(theta2 + theta3) - 1.39097218997047e-17*cos(theta3)^2 + 7.22223729145213e-35*cos(theta3)*cos(theta2 + theta3)^3 - 7.7763281472e-19*cos(theta3)*cos(theta2 + theta3)^2 + 1.54074395550979e-33*cos(theta3)*cos(theta2 + theta3) + 5.99785309872e-18*cos(theta3) - 8.640364608e-19*cos(theta2 + theta3)^3 - 7.480858836816e-18*cos(theta2 + theta3)^2 + 6.6642812208e-18*cos(theta2 + theta3) + 5.7699587139516e-17) + (-9.0e-5*(D_THETA_1^2)*sin(theta2) - 1.71e-5*(D_THETA_1^2)*sin(theta2 + theta3) + 3.078e-5*D_THETA_1*D_THETA_3*sin(theta3) + 3.078e-5*D_THETA_2*D_THETA_3*sin(theta3) + 1.539e-5*(D_THETA_3^2)*sin(theta3) - 0.005*F3 + 0.005*F4 - 0.008829*cos(theta1 + theta2) - 0.00167751*cos(theta1 + theta2 + theta3))*(-2.49317999999999e-13*cos(theta2)^2*cos(theta3) + 2.7702e-13*cos(theta2)^2*cos(theta2 + theta3) - 1.842183e-13*cos(theta2)^2 - 4.26333779999993e-14*cos(theta2)*cos(theta3)^2 + 4.73704200000003e-14*cos(theta2)*cos(theta3)*cos(theta2 + theta3) - 9.91059133949999e-13*cos(theta2)*cos(theta3) + 1.052676e-13*cos(theta2)*cos(theta2 + theta3)^2 + 6.866430615e-13*cos(theta2)*cos(theta2 + theta3) - 7.09006600102498e-13*cos(theta2) + 8.10034182e-15*cos(theta3)^2*cos(theta2 + theta3) - 9.39513330000007e-14*cos(theta3)^2 + 1.80007596e-14*cos(theta3)*cos(theta2 + theta3)^2 + 1.90108460835e-14*cos(theta3)*cos(theta2 + theta3) - 9.73235184075e-13*cos(theta3) + 1.0000422e-14*cos(theta2 + theta3)^3 + 1.37112462315e-13*cos(theta2 + theta3)^2 + 3.60344240460001e-13*cos(theta2 + theta3) - 6.67819295596249e-13)/(-1.6579647e-17*cos(theta2)^3 + 1.15555796663234e-33*cos(theta2)^2*cos(theta3)^2 + 8.5266756e-18*cos(theta2)^2*cos(theta3)*cos(theta2 + theta3) - 2.835119637e-18*cos(theta2)^2*cos(theta3) - 3.15013293e-18*cos(theta2)^2*cos(theta2 + theta3) - 2.7273964509225e-17*cos(theta2)^2 + 1.432159833059e-34*cos(theta2)*cos(theta3)^3 + 1.4580615276e-18*cos(theta2)*cos(theta3)^2*cos(theta2 + theta3) - 8.45561997e-18*cos(theta2)*cos(theta3)^2 + 1.620068364e-18*cos(theta2)*cos(theta3)*cos(theta2 + theta3)^2 + 1.402661031903e-17*cos(theta2)*cos(theta3)*cos(theta2 + theta3) + 3.08148791101958e-33*cos(theta2)*cos(theta3) - 4.54756032e-18*cos(theta2)*cos(theta2 + theta3)^2 + 3.507516432e-17*cos(theta2) + 2.17688294624968e-35*cos(theta3)^3*cos(theta2 + theta3) - 1.44591101487e-18*cos(theta3)^3 + 9.62964972193618e-35*cos(theta3)^2*cos(theta2 + theta3)^2 - 1.6065677943e-18*cos(theta3)^2*cos(theta2 + theta3) - 1.39097218997047e-17*cos(theta3)^2 + 7.22223729145213e-35*cos(theta3)*cos(theta2 + theta3)^3 - 7.7763281472e-19*cos(theta3)*cos(theta2 + theta3)^2 + 1.54074395550979e-33*cos(theta3)*cos(theta2 + theta3) + 5.99785309872e-18*cos(theta3) - 8.640364608e-19*cos(theta2 + theta3)^3 - 7.480858836816e-18*cos(theta2 + theta3)^2 + 6.6642812208e-18*cos(theta2 + theta3) + 5.7699587139516e-17) + (2.49317999999999e-13*cos(theta2)^2*cos(theta3) - 2.52435489670724e-29*cos(theta2)^2*cos(theta2 + theta3) + 1.842183e-13*cos(theta2)^2 + 4.26333779999993e-14*cos(theta2)*cos(theta3)^2 + 6.31088724176809e-30*cos(theta2)*cos(theta3)*cos(theta2 + theta3) + 4.4163613395e-13*cos(theta2)*cos(theta3) - 2.30937723e-13*cos(theta2)*cos(theta2 + theta3) + 3.030440501025e-13*cos(theta2) - 8.10034182e-15*cos(theta3)^2*cos(theta2 + theta3) - 9.0003798e-15*cos(theta3)*cos(theta2 + theta3)^2 - 1.234012160835e-13*cos(theta3)*cos(theta2 + theta3) - 5.05284480000003e-14*cos(theta2 + theta3)^2 - 4.37477124959999e-13*cos(theta2 + theta3) + 2.52435489670724e-29)*(0.00018*D_THETA_1*D_THETA_2*sin(theta2) + 3.42e-5*D_THETA_1*D_THETA_2*sin(theta2 + theta3) + 3.078e-5*D_THETA_1*D_THETA_3*sin(theta3) + 3.42e-5*D_THETA_1*D_THETA_3*sin(theta2 + theta3) + 9.0e-5*(D_THETA_2^2)*sin(theta2) + 1.71e-5*(D_THETA_2^2)*sin(theta2 + theta3) + 3.078e-5*D_THETA_2*D_THETA_3*sin(theta3) + 3.42e-5*D_THETA_2*D_THETA_3*sin(theta2 + theta3) + 1.539e-5*(D_THETA_3^2)*sin(theta3) + 1.71e-5*(D_THETA_3^2)*sin(theta2 + theta3) - 0.005*F1 + 0.005*F2 - 0.018639*cos(theta1) - 0.008829*cos(theta1 + theta2) - 0.00167751*cos(theta1 + theta2 + theta3))/(-1.6579647e-17*cos(theta2)^3 + 1.15555796663234e-33*cos(theta2)^2*cos(theta3)^2 + 8.5266756e-18*cos(theta2)^2*cos(theta3)*cos(theta2 + theta3) - 2.835119637e-18*cos(theta2)^2*cos(theta3) - 3.15013293e-18*cos(theta2)^2*cos(theta2 + theta3) - 2.7273964509225e-17*cos(theta2)^2 + 1.432159833059e-34*cos(theta2)*cos(theta3)^3 + 1.4580615276e-18*cos(theta2)*cos(theta3)^2*cos(theta2 + theta3) - 8.45561997e-18*cos(theta2)*cos(theta3)^2 + 1.620068364e-18*cos(theta2)*cos(theta3)*cos(theta2 + theta3)^2 + 1.402661031903e-17*cos(theta2)*cos(theta3)*cos(theta2 + theta3) + 3.08148791101958e-33*cos(theta2)*cos(theta3) - 4.54756032e-18*cos(theta2)*cos(theta2 + theta3)^2 + 3.507516432e-17*cos(theta2) + 2.17688294624968e-35*cos(theta3)^3*cos(theta2 + theta3) - 1.44591101487e-18*cos(theta3)^3 + 9.62964972193618e-35*cos(theta3)^2*cos(theta2 + theta3)^2 - 1.6065677943e-18*cos(theta3)^2*cos(theta2 + theta3) - 1.39097218997047e-17*cos(theta3)^2 + 7.22223729145213e-35*cos(theta3)*cos(theta2 + theta3)^3 - 7.7763281472e-19*cos(theta3)*cos(theta2 + theta3)^2 + 1.54074395550979e-33*cos(theta3)*cos(theta2 + theta3) + 5.99785309872e-18*cos(theta3) - 8.640364608e-19*cos(theta2 + theta3)^3 - 7.480858836816e-18*cos(theta2 + theta3)^2 + 6.6642812208e-18*cos(theta2 + theta3) + 5.7699587139516e-17) ;

end
